simulink model "M2V5_Motor_FrequencyResponse_CSL"  (R2021a)
settings: Solver=FixedStepDiscrete  StartTime=0.0  StopTime=inf  FixedStep=.004  RelTol=1e-3  EnableMultiTasking=on
PostLoadFcn:
  | try,
  | codertarget.arduinobase.registry.setBaudRate(gcs,115200)
  | disp('baud rate set to 115200 for external mode hardware serial')
  | baudrate='set_to_115200'
  | catch
  | disp('baud rate setting not needed in this version')
  | end
InitFcn:
  | MotorParams.Vsupply=4.78;
  | MotorParams.Voffset=0;
  | MotorParams.EncCov=2*pi/1336;
libraries: arduinolib x2, simulink x1, MinSegLibrary_M2V5 x1
settings Model: SimulationMode=external  SILPILModeSetting=veronly  ExtModeTrigDuration=2  Creator=Alec  LastModifiedBy=William Lee
settings SolverCC: AlgebraicLoopSolver=TrustRegion
settings DataIOCC: LimitDataPoints=on  SaveFormat=Array  ReturnWorkspaceOutputs=off
settings OptimizationCC: EnhancedBackFolding=on  PassReuseOutputArgsThreshold=0  ExpressionDepthLimit=2147483647  MaxStackSize=64  OptimizeBlockOrder=speed  DifferentSizesBufferReuse=on  OptimizationCustomize=off
settings DebuggingCC: UnderspecifiedInitializationDetection=Classic  MergeDetectMultiDrivingBlocksExec=none  ParameterTunabilityLossMsg=error  StateNameClashWarn=warning  SFUnexpectedBacktrackingDiag=warning  SFNoUnconditionalDefaultTransitionDiag=warning  SFExecutionAtInitializationDiag=none  SFMachineParentedDataDiag=warning  ArithmeticOperatorsInVariantConditions=warning
settings HardwareCC: ProdBitPerInt=16  ProdBitPerPointer=16  ProdBitPerSizeT=16  ProdBitPerPtrDiffT=16  ProdLargestAtomicFloat=None  ProdWordSize=8  ProdHWDeviceType=Atmel->AVR  UseEmbeddedCoderFeatures=off  UseSimulinkCoderFeatures=off
settings ModelReferenceCC: PropagateSignalLabelsOutOfModel=off
settings SFSimCC: SimUseLocalCustomCode=off  MATLABDynamicMemAlloc=off  CustomCodeUndefinedFunction=UseInterfaceOnly
settings RTWCC: SystemTargetFile=ert.tlc  HardwareBoard=Arduino Mega 2560  TemplateMakefile=ert_default_tmf  GenerateReport=on  RTWVerbose=off  RTWUseLocalCustomCode=off  Toolchain=Arduino AVR  BuildConfiguration=Faster Runs  LaunchReport=on
settings CodeAppCC: ForceParamTrailComments=on  OperatorAnnotations=on
settings ERTTargetCC: ERTCustomFileBanners=off  SupportContinuousTime=on  SupportNonInlinedSFcns=on  RemoveResetFunc=off  SupportVariableSizeSignals=on  ModelStepFunctionPrototypeControlCompliant=off  ExtModeStaticAllocSize=2048
settings ConfigComp: CovMetricSettings=dw  CovSaveCumulativeToWorkspaceVar=on  CovSaveSingleToWorkspaceVar=on  CovExternalEMLEnable=off

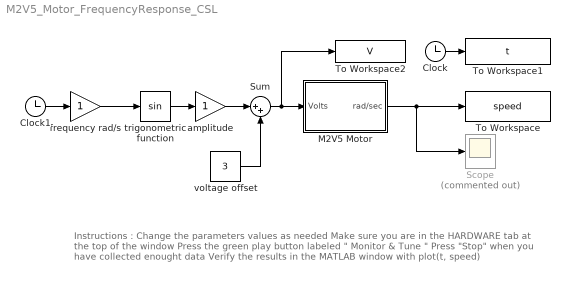
== system M2V5_Motor_FrequencyResponse_CSL ==
  note: Instructions :
      |
      | Change the parameters values as needed
      | Make sure you are in the HARDWARE tab at the top of the window
      | Press the green play button labeled " Monitor & Tune "
      | Press "Stop" when you have collected enought data
      | Verify the results in the MATLAB window with plot(t, speed)
  Clock : Clock
  Clock1 : Clock
  M2V5 Motor : Subsystem
  Scope : Scope  Commented=on
  Sum : Sum  Inputs=|++
  To Workspace : ToWorkspace  VariableName=speed  SampleTime=-1
      settings: Save2DSignal=2-D array (concatenate along first dimension)
  To Workspace1 : ToWorkspace  VariableName=t  SampleTime=-1
      settings: Save2DSignal=2-D array (concatenate along first dimension)
  To Workspace2 : ToWorkspace  VariableName=V  SampleTime=-1
      settings: Save2DSignal=2-D array (concatenate along first dimension)
  amplitude : Gain
  "frequency rad/s " : Gain
  "trigonometric function " : Trigonometry
  "voltage offset " : Constant  Value=3
  wires:
  Clock/1 -> To Workspace1/1
  M2V5 Motor/1(rad/sec) -> Scope/1, To Workspace/1
  Clock1/1 -> "frequency rad/s "/1
  "frequency rad/s "/1 -> "trigonometric function "/1
  "trigonometric function "/1 -> amplitude/1
  amplitude/1 -> Sum/1
  "voltage offset "/1 -> Sum/2
  Sum/1 -> To Workspace2/1, M2V5 Motor/1(Volts)

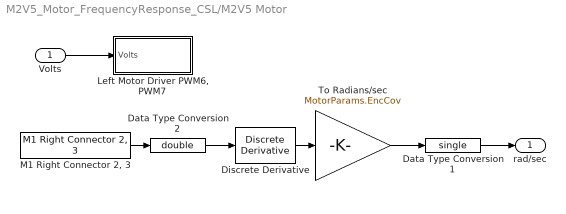
== system M2V5_Motor_FrequencyResponse_CSL/M2V5 Motor ==
  Volts : Inport
  Data Type Conversion1 : DataTypeConversion  OutDataTypeStr=single
  Data Type Conversion2 : DataTypeConversion  OutDataTypeStr=double
  Discrete Derivative : simulink/Discrete/Discrete Derivative  gainval=1.0  ICPrevScaledInput=0.0  OutMin=[]  OutMax=[]  OutDataType=fixdt(1, 16)  OutScaling=2^-10  DoSatur=off
  "Left Motor Driver PWM6, PWM7" : Subsystem  mask{Vsupply=MotorParams.Vsupply, Voffset=MotorParams.Voffset}
      mask prompts: Vsupply "Driver Voltage"; Voffset "Voltage offset (0-Vsupply)"
      mask help:
      | Specify driver supply voltage (3.9 for USB)
      | Specify the PWM offset (0-255)
      mask Display:
      | port_label('input',1,'Volts')
      | text(15,5,['Vsupply=' num2str(Vsupply)])
  "M1 Right Connector 2, 3" : MinSegLibrary_M2V5/M1 Right Connector 2, 3  Encoder=0  PinA=2  PinB=3
      settings: SourceProductName=Rensselaer Arduino Support Package
  To Radians/sec : Gain  Gain=MotorParams.EncCov
  rad/sec : Outport
  wires:
  Discrete Derivative/1 -> To Radians/sec/1
  To Radians/sec/1 -> Data Type Conversion1/1
  "M1 Right Connector 2, 3"/1 -> Data Type Conversion2/1
  Data Type Conversion2/1 -> Discrete Derivative/1
  Data Type Conversion1/1 -> rad/sec/1
  Volts/1 -> "Left Motor Driver PWM6, PWM7"/1(Volts)

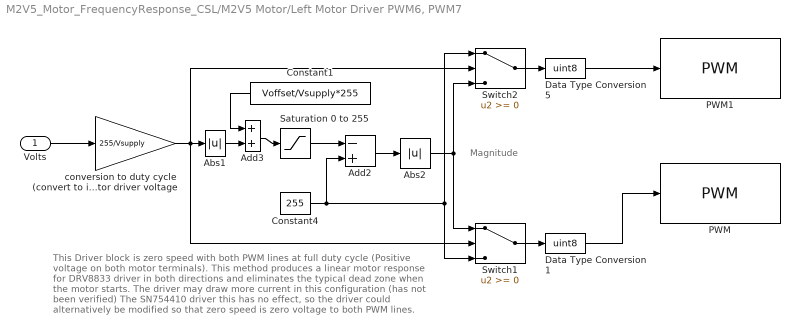
== system M2V5_Motor_FrequencyResponse_CSL/M2V5 Motor/Left Motor Driver PWM6, PWM7 ==
  note: Magnitude
  note: This Driver block is zero speed with both PWM lines at full duty cycle
      |  (Positive voltage on both motor terminals).
      | This method produces a linear motor response for DRV8833 driver
      |  in both directions and eliminates
      | the typical dead zone when the motor starts.
      | The driver may draw more current in this configuration (has not been verified)
      |
      | The SN754410 driver this has no effect, so the driver could alternatively
      | be modified so that zero speed is zero voltage to both PWM lines.
  Volts : Inport
  Abs1 : Abs
  Abs2 : Abs
  Add2 : Sum  Inputs=-+
  Add3 : Sum
  Constant1 : Constant  Value=Voffset/Vsupply*255
  Constant4 : Constant  Value=255
  Data Type Conversion1 : DataTypeConversion  OutDataTypeStr=uint8
  Data Type Conversion5 : DataTypeConversion  OutDataTypeStr=uint8
  PWM : arduinolib/PWM  pinNumber=7  frequencyType=Default  desiredFrequency=490.2  achievableFrequency=490.2
  PWM1 : arduinolib/PWM  pinNumber=6  frequencyType=Default  desiredFrequency=490.2  achievableFrequency=490.2
  Saturation 0 to 255 : Saturate  UpperLimit=255  LowerLimit=0
  Switch1 : Switch
  Switch2 : Switch
  conversion to duty cycle (convert to int) denominator is motor driver voltage : Gain  Gain=255/Vsupply  OutDataTypeStr=int16
  wires:
  Data Type Conversion1/1 -> PWM/1
  Data Type Conversion5/1 -> PWM1/1
  Switch1/1 -> Data Type Conversion1/1
  Switch2/1 -> Data Type Conversion5/1
  Abs2/1 -> Switch1/1, Switch2/3
  Add2/1 -> Abs2/1
  Constant4/1 -> Add2/2, Switch2/1, Switch1/3
  Saturation 0 to 255/1 -> Add2/1
  conversion to duty cycle (convert to int) denominator is motor driver voltage/1 -> Abs1/1, Switch2/2, Switch1/2
  Abs1/1 -> Add3/2
  Constant1/1 -> Add3/1
  Add3/1 -> Saturation 0 to 255/1
  Volts/1 -> conversion to duty cycle (convert to int) denominator is motor driver voltage/1
